simulink model "TRIAD"  (R2017a)
settings: Solver=ode4  StartTime=0.0  StopTime=20000  FixedStep=0.1  RelTol=1e-3  EnableMultiTasking=on
undefined symbols (not defined in the file): mbaseserialmask, RxBuffer
libraries: xpcseriallib x17, vrlib x7, slrtlib x4, sharedtransform x3, sharedutil x2, dspinverses x2, dspmathops x2, simulink x1, dspsigops x1
(part 2 of 3)

== system TRIAD/Subsystem/Comm and data set/Packet ZOH ==
  note: Packet Size = 22
      | =============
      | Header: 2Byte
      | Length: 1Byte
      | Time: 4 Bytes (Float32)
      | torqueX: 2Byte
      | torqueY: 2Byte
      | torqueZ: 2Byte
      | Roll      : 2Byte
      | Pitch    : 2Byte
      | Yaw     : 2Byte
      | dummy: 1byte
      | CRC: 2Byte
      | =============
  packet _count : Inport
  Data Store Write1 : DataStoreWrite  DataStoreName=RxBuffer  DataStoreElements=RxBuffer(:)
  If1 : If
  Merge1 : Merge
  No packet received Use buffer value : Subsystem  TreatAsAtomicUnit=on
  Select Main Packet : Selector  InputPortWidth=23  IndexOptions=Index vector (dialog)  Indices=[2:23]  OutputSizes=1
  Select Packet Size : Selector  InputPortWidth=23  IndexOptions=Index vector (dialog)  Indices=[1]  OutputSizes=1
  UDP Memory1 : DataStoreMemory  DataStoreName=RxBuffer  ReadBeforeWriteMsg=warning  WriteAfterWriteMsg=warning  WriteAfterReadMsg=warning  VectorParams1D=off  ShowAdditionalParam=off  Dimensions=22
  Valid Packet (Bypass) : Subsystem  TreatAsAtomicUnit=on
  packet : Outport
  wires:
  Select Main Packet/1 -> Valid Packet (Bypass)/1(In1)
  Select Packet Size/1 -> If1/1
  packet _count/1 -> Select Packet Size/1, Select Main Packet/1
  Valid Packet (Bypass)/1(Out1) -> Merge1/1
  Merge1/1 -> Data Store Write1/1, packet/1
  If1/2 -> No packet received Use buffer value/Action
  No packet received Use buffer value/1(Out1) -> Merge1/2
  If1/1 -> Valid Packet (Bypass)/Action

== system TRIAD/Subsystem10/Subsystem7/eular rotational equation2 ==
  Torque : Inport
  Inertial : Inport  Port=2
  omega_0 : Inport  Port=3
  " LU Inverse" : dspinverses/ LU Inverse
      settings: SourceProductName=DSP System Toolbox
  Cross Product : vrlib/Utilities/Cross Product
      settings: SourceProductBaseCode=VR
  Integrator1 : Integrator  InitialConditionSource=external
  Matrix Multiply : Product  Multiplication=Matrix(*)
  Matrix Multiply1 : Product  Multiplication=Matrix(*)
  Sum : Sum  Inputs=|-+
  omega : Outport
  omega_dot : Outport  Port=2
  wires:
  omega_0/1 -> Integrator1/2
  Matrix Multiply1/1 -> Integrator1/1, omega_dot/1
  Matrix Multiply/1 -> Cross Product/2
  Cross Product/1 -> Sum/1
  Torque/1 -> Sum/2
  Inertial/1 -> Matrix Multiply/1, " LU Inverse"/1
  Integrator1/1 -> Cross Product/1, Matrix Multiply/2, omega/1
  " LU Inverse"/1 -> Matrix Multiply1/1
  Sum/1 -> Matrix Multiply1/2

== system TRIAD/Subsystem10/Subsystem8/Kinematics (quaternion2)1 ==
  quat : Inport
  omega : Inport  Port=2
  Gain : Gain  Gain=0.5  SaturateOnIntegerOverflow=on  OutDataTypeStr=Inherit: Same as input  ParamDataTypeStr=Inherit: Same as input
  Mux1 : Mux  Inputs=2
  Mux2 : Mux
  q1dot : Fcn  Expr=-u(2)*u(5) - u(3)*u(6) - u(4)*u(7)
  q2dot : Fcn  Expr=u(1)*u(5) + u(3)*u(7) - u(4)*u(6)
  q3dot : Fcn  Expr=u(1)*u(6) - u(2)*u(7) + u(4)*u(5)
  q4dot : Fcn  Expr=u(1)*u(7) + u(2)*u(6) - u(3)*u(5)
  quat2dot : Outport
  wires:
  Mux2/1 -> Gain/1
  Mux1/1 -> q1dot/1, q2dot/1, q4dot/1, q3dot/1
  q1dot/1 -> Mux2/1
  q2dot/1 -> Mux2/2
  q3dot/1 -> Mux2/3
  q4dot/1 -> Mux2/4
  Gain/1 -> quat2dot/1
  quat/1 -> Mux1/1
  omega/1 -> Mux1/2

== system TRIAD/Subsystem10/Subsystem8/quat to Euler1 ==
  quat : Inport
  Mux : Mux  Inputs=3
  phi : Fcn  Expr=atan2( 2*(u(3)*u(4) + u(1)*u(2)) , u(1)^2 - u(2)^2 - u(3)^2 + u(4)^2 )
  psi : Fcn  Expr=atan2( 2*(u(2)*u(3) + u(1)*u(4)) , u(1)^2 + u(2)^2 - u(3)^2 - u(4)^2 )
  theta : Fcn  Expr=asin(2*(u(1)*u(3) - u(2)*u(4)))
  euler : Outport
  wires:
  Mux/1 -> euler/1
  phi/1 -> Mux/1
  theta/1 -> Mux/2
  psi/1 -> Mux/3
  quat/1 -> psi/1, phi/1, theta/1

== system TRIAD/Subsystem9/Subsystem7/eular rotational equation2 ==
  Torque : Inport
  Inertial : Inport  Port=2
  omega_0 : Inport  Port=3
  " LU Inverse" : dspinverses/ LU Inverse
      settings: SourceProductName=DSP System Toolbox
  Cross Product : vrlib/Utilities/Cross Product
      settings: SourceProductBaseCode=VR
  Integrator1 : Integrator  InitialConditionSource=external
  Matrix Multiply : Product  Multiplication=Matrix(*)
  Matrix Multiply1 : Product  Multiplication=Matrix(*)
  Sum : Sum  Inputs=|-+
  omega : Outport
  omega_dot : Outport  Port=2
  wires:
  omega_0/1 -> Integrator1/2
  Matrix Multiply1/1 -> Integrator1/1, omega_dot/1
  Matrix Multiply/1 -> Cross Product/2
  Cross Product/1 -> Sum/1
  Torque/1 -> Sum/2
  Inertial/1 -> Matrix Multiply/1, " LU Inverse"/1
  Integrator1/1 -> Cross Product/1, Matrix Multiply/2, omega/1
  " LU Inverse"/1 -> Matrix Multiply1/1
  Sum/1 -> Matrix Multiply1/2

== system TRIAD/Subsystem9/Subsystem8/Kinematics (quaternion2)1 ==
  quat : Inport
  omega : Inport  Port=2
  Gain : Gain  Gain=0.5  SaturateOnIntegerOverflow=on  OutDataTypeStr=Inherit: Same as input  ParamDataTypeStr=Inherit: Same as input
  Mux1 : Mux  Inputs=2
  Mux2 : Mux
  q1dot : Fcn  Expr=-u(2)*u(5) - u(3)*u(6) - u(4)*u(7)
  q2dot : Fcn  Expr=u(1)*u(5) + u(3)*u(7) - u(4)*u(6)
  q3dot : Fcn  Expr=u(1)*u(6) - u(2)*u(7) + u(4)*u(5)
  q4dot : Fcn  Expr=u(1)*u(7) + u(2)*u(6) - u(3)*u(5)
  quat2dot : Outport
  wires:
  Mux2/1 -> Gain/1
  Mux1/1 -> q1dot/1, q2dot/1, q4dot/1, q3dot/1
  q1dot/1 -> Mux2/1
  q2dot/1 -> Mux2/2
  q3dot/1 -> Mux2/3
  q4dot/1 -> Mux2/4
  Gain/1 -> quat2dot/1
  quat/1 -> Mux1/1
  omega/1 -> Mux1/2

== system TRIAD/Subsystem9/Subsystem8/quat to Euler1 ==
  quat : Inport
  Mux : Mux  Inputs=3
  phi : Fcn  Expr=atan2( 2*(u(3)*u(4) + u(1)*u(2)) , u(1)^2 - u(2)^2 - u(3)^2 + u(4)^2 )
  psi : Fcn  Expr=atan2( 2*(u(2)*u(3) + u(1)*u(4)) , u(1)^2 + u(2)^2 - u(3)^2 - u(4)^2 )
  theta : Fcn  Expr=asin(2*(u(1)*u(3) - u(2)*u(4)))
  euler : Outport
  wires:
  Mux/1 -> euler/1
  phi/1 -> Mux/1
  theta/1 -> Mux/2
  psi/1 -> Mux/3
  quat/1 -> psi/1, phi/1, theta/1

== system TRIAD/Subsystem/Comm and data set/Baseboard Serial/RS232 ISR ==
  Xmt 1 : Inport
  Xmt 2 : Inport  Port=2
  function : TriggerPort  TriggerType=function-call  VariantControl=Variant
  Demux : Demux
  Read Int Status FC1 : xpcseriallib/Mainboard/Baseboard Serial Internal  blocks/Read Int Status FC  addr1=baddr1  addr2=baddr2
      settings: SourceProductName=Simulink Real-Time  SourceProductBaseCode=XP
  Receive 1 : Subsystem  TreatAsAtomicUnit=on
  Receive 2 : Subsystem  TreatAsAtomicUnit=on
  Transmit 1 : Subsystem  TreatAsAtomicUnit=on
  Transmit 2 : Subsystem  TreatAsAtomicUnit=on
  Recv 1 : Outport
  Recv 2 : Outport  Port=2
  wires:
  Receive 1/1(Recv 1) -> Recv 1/1
  Xmt 1/1 -> Transmit 1/1(Xmt 1)
  Receive 2/1(Recv 2) -> Recv 2/1
  Xmt 2/1 -> Transmit 2/1(Xmt 2)
  Read Int Status FC1/1 -> Demux/1
  Demux/1 -> Receive 1/Trigger
  Demux/4 -> Transmit 2/Trigger
  Demux/3 -> Receive 2/Trigger
  Demux/2 -> Transmit 1/Trigger
  Read Int Status FC1/2 -> Transmit 1/2(Enable), Transmit 2/2(Enable)

== system TRIAD/Subsystem/Comm and data set/Packet ZOH/No packet received Use buffer value ==
  Action Port : ActionPort  ActionType=else
  Data Store Read : DataStoreRead  DataStoreName=RxBuffer  DataStoreElements=RxBuffer(:)
  Out1 : Outport
  wires:
  Data Store Read/1 -> Out1/1

== system TRIAD/Subsystem/Comm and data set/Packet ZOH/Valid Packet (Bypass) ==
  In1 : Inport
  Action Port : ActionPort  ActionType=then
  Out1 : Outport
  wires:
  In1/1 -> Out1/1

== system TRIAD/Subsystem/Comm and data set/Baseboard Serial/RS232 ISR/Receive 1 ==
  function : TriggerPort  TriggerType=function-call  VariantControl=Variant
  Constant : Constant  OutDataTypeStr=uint32
  FIFO write 1 : xpcseriallib/FIFO write   size=1024  inputtype=count+32 bit uint  present=off  sampletime=-1  id=RCV channel 1, IRQ 4
      settings: SourceProductName=Simulink Real-Time  SourceProductBaseCode=XP
  Read HW FIFO1 : xpcseriallib/Mainboard/Baseboard Serial Internal  blocks/Read HW FIFO  flush=on  addr=baddr1
      settings: SourceProductName=Simulink Real-Time  SourceProductBaseCode=XP
  Recv 1 : Outport
  wires:
  Read HW FIFO1/1 -> FIFO write 1/1
  FIFO write 1/1 -> Recv 1/1
  Constant/1 -> Read HW FIFO1/1

== system TRIAD/Subsystem/Comm and data set/Baseboard Serial/RS232 ISR/Receive 2 ==
  function : TriggerPort  TriggerType=function-call  VariantControl=Variant
  Constant : Constant  OutDataTypeStr=uint32
  FIFO write 2 : xpcseriallib/FIFO write   size=1024  inputtype=count+32 bit uint  present=off  sampletime=-1  id=RCV channel 2, IRQ 4
      settings: SourceProductName=Simulink Real-Time  SourceProductBaseCode=XP
  Read HW FIFO2 : xpcseriallib/Mainboard/Baseboard Serial Internal  blocks/Read HW FIFO  flush=on  addr=baddr2
      settings: SourceProductName=Simulink Real-Time  SourceProductBaseCode=XP
  Recv 2 : Outport
  wires:
  Read HW FIFO2/1 -> FIFO write 2/1
  FIFO write 2/1 -> Recv 2/1
  Constant/1 -> Read HW FIFO2/1

== system TRIAD/Subsystem/Comm and data set/Baseboard Serial/RS232 ISR/Transmit 1 ==
  Xmt 1 : Inport
  Enable : Inport  Port=2
  function : TriggerPort  TriggerType=function-call  VariantControl=Variant
  Constant1 : Constant  OutDataTypeStr=uint32
  FIFO read 1 : xpcseriallib/FIFO read   maxsize=60  minsize=1  usedelimiter=off  delimiter=13  outputtype=count+32 bit uint  enable=on  enableout=on  sampletime=-1
      settings: SourceProductName=Simulink Real-Time  SourceProductBaseCode=XP
  Write HW FIFO1 : xpcseriallib/Mainboard/Baseboard Serial Internal  blocks/Write HW FIFO  addr=baddr1
      settings: SourceProductName=Simulink Real-Time  SourceProductBaseCode=XP
  wires:
  Constant1/1 -> FIFO read 1/3
  FIFO read 1/2 -> Write HW FIFO1/2
  FIFO read 1/1 -> Write HW FIFO1/1
  Xmt 1/1 -> FIFO read 1/1
  Enable/1 -> FIFO read 1/2

== system TRIAD/Subsystem/Comm and data set/Baseboard Serial/RS232 ISR/Transmit 2 ==
  Xmt 2 : Inport
  Enable : Inport  Port=2
  function : TriggerPort  TriggerType=function-call  VariantControl=Variant
  Constant2 : Constant  OutDataTypeStr=uint32
  FIFO read 2 : xpcseriallib/FIFO read   maxsize=60  minsize=1  usedelimiter=off  delimiter=13  outputtype=count+32 bit uint  enable=on  enableout=on  sampletime=-1
      settings: SourceProductName=Simulink Real-Time  SourceProductBaseCode=XP
  Write HW FIFO2 : xpcseriallib/Mainboard/Baseboard Serial Internal  blocks/Write HW FIFO  addr=baddr2
      settings: SourceProductName=Simulink Real-Time  SourceProductBaseCode=XP
  wires:
  Constant2/1 -> FIFO read 2/3
  FIFO read 2/2 -> Write HW FIFO2/2
  FIFO read 2/1 -> Write HW FIFO2/1
  Enable/1 -> FIFO read 2/2
  Xmt 2/1 -> FIFO read 2/1

== matlab function TRIAD/Subsystem5/Keplerian Differential Equation ==
  data: kepel input; deltakep output
function deltakep  = delkep(kepel)
% [deltakep] = delkep (kep_el)
%	Function delkep calculates the rate of
%	variation of keplerian elements, considering only
%	J2 and J4.
%
% Input:
%	kep_el
% 		vector with the keplerian elements:
%		(1) - semimajor axis of the orbit in meters.
%		(2) - eccentricity.
%		(3) - inclination in radians.
%		(4) - right ascension of ascending node in radians.
%		(5) - argument of perigee in radians.
%		(6) - mean anomaly in radians.
%       Obs: 4,5 and 6 are not used
%
% Output:
%	deltakep
%		(1) = 0
%		(2) = 0
%		(3) = 0
%		(4) - variation rate of the right ascension of
%		      ascending node, in radians/second.
%		(5) - variation rate of the argument of perigee,
%			  in radians/second.
%		(6) - variation rate of the mean anomaly, in
%			  radians/second.
%
% Authors:
%	Valder M. de Medeiros  	september/81 	version 1.0
%	Valdemir Carrara 		july 2005		(C Version)
%   Valdemir Carrara            March/09        Matlab

EARTH_RADIUS	= 6378139.;				% Earth's radius in meters
EARTH_GRAVITY	= 3.9860064e+14;		% Earth's gravitational constant (m**3/s**2)
J_2 			=  1.0826268362e-3;		% = 484.16544e-6 * SQRT(5.e0)
J_4 			= -1.62336e-6;			% = -0.54112e-6 * 3e0

seix = kepel(1);
exce = kepel(2);
exc2 = exce*exce;
eta2 = 1. - exc2;
eta1 = sqrt(eta2);
teta = cos(kepel(3));
tet2 = teta*teta;
tet4 = tet2*tet2;
aux0 = sqrt(EARTH_GRAVITY/(seix*seix*seix));
plar = EARTH_RADIUS/(seix*eta2);
pla2 = plar*plar;
gam2 = 0.5*J_2*pla2;
gam4 = -0.375*J_4*pla2*pla2;

deltakep = [0, 0, 0, 0, 0, 0];

deltakep(4) = aux0*teta*(3.*gam2*(-1. + 0.125*gam2*(9.*eta2 + 12.*eta1 - ...
	   5. - (5.*eta2 + 36.*eta1 + 35.)*tet2)) + ...
	   1.25*gam4*(5. - 3.*eta2)*(3. - 7.*tet2));
deltakep(5) = aux0*(1.5*gam2*((5.*tet2 - 1.) + ...
	   0.0625*gam2*(25.*eta2 + 24.*eta1 - ...
	   35. + (90. - 192.*eta1 - 126.*eta2)*tet2 + ...
	   (385. + 360.*eta1 + 45.*eta2)*tet4)) + ...
	   0.3125*gam4*(21. - 9.*eta2 + (-270. + 126.*eta2)*tet2 + ...
	   (385. - 189.*eta2)*tet4));
deltakep(6) = aux0*(1. + eta1*(1.5*gam2*((3.*tet2 - 1.) + ...
	   0.0625*gam2*(16.*eta1 + 25.*eta2 - 15. + ...
	   (30. - 96.*eta1 - 90.*eta2)*tet2 + ...
	   (105. + 144.*eta1 + 25.*eta2)*tet4)) + ...
	   0.9375*gam4*exc2*(3. - 30.*tet2 + 35.*tet4)));

== matlab function TRIAD/Subsystem2/Convert Keplerian parameters to states ==
  data: kepel input; statvec output
function statvec = kepel_statvec(kepel)
%  [statvec] = kepel_statvec (kepel)
%	The function kepel_statvec transforms the keplerian
%	elements kepel into the corresponding state vector in
%	the same reference system.
%
% Input:
%	kepel
% 		vector containing the keplerian elements:
%		(1) - semimajor axis of the orbit in meters.
%		(2) - eccentricity.
%		(3) - inclination in radians.
%		(4) - right ascension of ascending node in radians.
%		(5) - argument of perigee in radians.
%		(6) - mean anomaly in radians.
%
% Output:
%	statvec
%  		state vector in meters and meters/second.
%
% Authors:
%	Helio K. Kuga;
%	Valder M. Medeiros;
%	Valdemir Carrara		february/80		version 1.0
%	Valdemir Carrara		july 2005		(C version)
%   Valdemir Carrara            March/09        Matlab

EARTH_GRAVITY	= 3.9860064e+14;		% Earth's gravitational constant (m**3/s**2)

a    = kepel(1);	% semi-major axis
exc  = kepel(2);	% eccentricity

c1   = sqrt(1. - exc*exc);

% Rotational matrix
rot_maz1 =  [cos(-kepel(4)), sin(-kepel(4)), 0;
             -sin(-kepel(4)), cos(-kepel(4)), 0; 
             0, 0, 1];
         
rot_max =  [1, 0, 0; 
           0, cos(-kepel(3)), sin(-kepel(3));
           0, -sin(-kepel(3)), cos(-kepel(3))];
       
rot_maz2 =  [cos(-kepel(5)), sin(-kepel(5)), 0;
             -sin(-kepel(5)), cos(-kepel(5)), 0; 
             0, 0, 1];
         
orb2iner = rot_maz1*rot_max*rot_maz2;

%%%%%%%%%%%%%%%%%%%%%%%%%%%%%%%%%%%%%%%%%%%%
%     Kepler's equation
%E    = kepler(kepel(6), exc);
mean_anomaly = kepel(6);
eccentricity = exc;
%function [eccentric] = kepler (mean_anomaly, eccentricity)
% [eccentric] = kepler (mean_anomaly, eccentricity)
%	The subroutine kepler finds a solution to the
%	kepler's equation.
%
% Input:
%	mean_anomaly
%		mean anomaly in radians.
%	eccentricity
%		eccentricity.
%
% Output:
%	eccentric
%		eccentric anomaly in radians.
%
% Authors:
%	Valder M. de Medeiros		june/81		version 2.0
%	Valdemir Carrara			july 2005	(C version)
%   Valdemir Carrara            March/09        Matlab

exc2    = eccentricity*eccentricity;
am1     = mod (mean_anomaly, 2*pi);
am2     = am1 + am1;
am3     = am1 + am2;
shoot   = am1 + eccentricity*(1. - 0.125*exc2)*sin(am1) + ...
		0.5*exc2*(sin(am2) + 0.75*eccentricity*sin(am3));
shoot   = mod (shoot, 2*pi);

e1      = 1.0;
ic      = 0;

while ((abs(e1) > 1.e-12) && (ic <= 10)) 
	e1    = (shoot - am1 - eccentricity*sin(shoot)) / ...
			(1.0 - eccentricity*cos(shoot));
    shoot = shoot - e1;
    ic    = ic + 1;
end

if (ic >= 10)
    disp ('warning ** subroutine kepler did not converge in 10 iterations');
end

%eccentric = shoot;
E = shoot;
%%%%%%%%%%%%%%%%%%%%%%%%%%%%%%%%%%%%%%%%%%%%%%
sE   = sin(E);
cE   = cos(E);
c3   = sqrt(EARTH_GRAVITY/a)/(1. - exc*cE);

%     state vector

statvec = [[a*(cE - exc), a*c1*sE, 0]*orb2iner', [-c3*sE, c1*c3*cE, 0]*orb2iner'];

== matlab function TRIAD/Ephemerides Date/Modified Julian Date (mjd) ==
  data: dmy input; diju output
function diju  =  djm (dmy)
% [diju] = djm (day, month, year)
%    The function djm furnishes the Modified Julian
%    Date with reference to the day, month and year,
%    at zero hours of the day.
% inputs:
%   dmy(1): day, day of the month
%   dmy(2): month, month of the year
%   dmy(3): year

% outputs:
%   diju
%       Modified Julian Date in days, referred to 1950.0. 
%
% Valdemir Carrara, Apr, 2003
%

diju = 367*dmy(3) + dmy(1) - 712269 + fix(275*dmy(2)/9)- fix(7*(dmy(3)+fix((dmy(2)+9)/12))/4);

== matlab function TRIAD/Ephemerides Date/Modified Julian Date (mjd0) ==
  data: dmy input; diju output
function diju  =  djm (dmy)
% [diju] = djm (day, month, year)
%    The function djm furnishes the Modified Julian
%    Date with reference to the day, month and year,
%    at zero hours of the day.
% inputs:
%   dmy(1): day, day of the month
%   dmy(2): month, month of the year
%   dmy(3): year

% outputs:
%   diju
%       Modified Julian Date in days, referred to 1950.0. 
%
% Valdemir Carrara, Apr, 2003
%

diju = 367*dmy(3) + dmy(1) - 712269 + fix(275*dmy(2)/9)- fix(7*(dmy(3)+fix((dmy(2)+9)/12))/4);

== matlab function TRIAD/Ephemerides Date/Modified Julian Date (mjd1) ==
  data: dmy input; diju output
function diju  =  djm (dmy)
% [diju] = djm (day, month, year)
%    The function djm furnishes the Modified Julian
%    Date with reference to the day, month and year,
%    at zero hours of the day.
% inputs:
%   dmy(1): day, day of the month
%   dmy(2): month, month of the year
%   dmy(3): year

% outputs:
%   diju
%       Modified Julian Date in days, referred to 1950.0. 
%
% Valdemir Carrara, Apr, 2003
%

diju = 367*dmy(3) + dmy(1) - 712269 + fix(275*dmy(2)/9)- fix(7*(dmy(3)+fix((dmy(2)+9)/12))/4);

== matlab function TRIAD/Ephemerides Time ==
  data: hours input; dayf output; minutes input; seconds input
function dayf  = time_to_dayf(hours, minutes, seconds)
% [dayf] = time_to_dayf (hours, minutes, seconds)
%    The function time_to_dayf returns with the day elapesed
%    time in seconds
% inputs:
%   hours     
%       day hour (integer).
%   minutes
%       minutes (integer).
%   seconds
%       seconds and fraction of second
% outputs:
%   dayf
%       Day elapsed time in seconds. 
%
% Valdemir Carrara, Feb, 2009
%

dayf = seconds + 60*(minutes + 60*hours);

== matlab function TRIAD/Subsystem9/MATLAB Function ==
  data: Magnetic_torque output; gyro input; Magnetic_torque input; flg output
function [Magnetic_torque, flg] = fcn(gyro, Magnetic_torque)

persistent stack_magx
persistent stack_magy
persistent stack_magz
persistent cnt_

if isempty(stack_magx)
    stack_magx = 0;
    stack_magy = 0;
    stack_magz = 0;
    cnt_ = 0;
else
    cnt_ = cnt_ + 1;
end

flg = 0;

if cnt_ >= 100
    if (abs(stack_magx)<0.1) && (abs(stack_magy)<0.1) && (abs(stack_magz)<0.1)
        flg = 1;
        Magnetic_torque = [0 0 0]';
    else
        flg = 0;
    end
    stack_magx = 0;
    stack_magy = 0;
    stack_magz = 0;
    cnt_ = 0;
else
    stack_magx = stack_magx + gyro(1);
    stack_magy = stack_magy + gyro(2);
    stack_magz = stack_magz + gyro(3);
end



end

== matlab function TRIAD/Subsystem2/ECI to ECEF  ==
  data: tesig input; xterrestrial output; xi input
function xterrestrial  = inertial_to_terrestrial (tesig, xi)
% [xterrestrial] = inertial_to_terrestrial (tesig, xi)
%	The function inertial_to_terrestrial transforms geocentric
%	inertial state vector into geocentric
%	terrestrial coordinates (referred to
%	Greenwich).
%
% Input:
%	tesig
%		Greenwich sidereal time in radians.
%	xi
%		geocentric inertial position vector.
%       (1) inertial geocentric position x (m)
%       (2) inertial geocentric position y (m)
%       (3) inertial geocentric position z (m)
%       (4) inertial geocentric velocity x (m/s)
%       (5) inertial geocentric velocity y (m/s)
%       (6) inertial geocentric velocity z (m/s)
%
% Output:
%	xterrestrial
%		corresponding geocentric terrestrial vector.
%
% Authors:
%	Helio/Valder/Valdemir-aug. 1981 - version 1.0
%	Helio		-july 1989 - version 1.1
%	Valdemir Carrara		july 2005		(C version)
%   Valdemir Carrara            March/09        Matlab
coan    =  cos(tesig);
sian    =  sin(tesig);
rot_mat =  [ coan, sian, 0 ;
            -sian, coan, 0 ; 
                0,    0, 1];

xterrestrial_ = [xi(1:3); xi(4:6)]*rot_mat';
xterrestrial  = [xterrestrial_(1,:) xterrestrial_(2,:)];

== matlab function TRIAD/Subsystem2/Convert Terrestrial Geocentric to Speherical coordinates ECEF2LLA ==
  data: geoc input; spherical output
function spherical  = rectangular_to_spherical (geoc)
% [spherical] = rectangular_to_spherical (geoc)
%	Function to transform rectangular terrestrial
%	geocentric coordinates in spherical coordinates
%	(longitude, geocentric latitude and distance).
%
% Inputs:
%   geoc
%   		geocentric rectangular coordinates vector in meters
%           (1) geocentric position x (m)
%           (2) geocentric position y (m)
%           (3) geocentric position z (m)
%
% Outputs:
%	spherical
%		Geocentric coordinates vector:
%			1 = east longitude (rad)
%			2 = geocentric latitude (rad)
%			3 = geocentric distance (meters)
%
% Authors:
%   Valdemir Carrara            May/09        Matlab

px = geoc(1);
py = geoc(2);
pz = geoc(3);
ws = px*px + py*py;
rw = sqrt(ws + pz *pz);
lg = atan2(py, px);
lt = atan2(pz, sqrt(ws));
spherical = [lg, lt, rw];

== matlab function TRIAD/Greenwich Aparent Mean Sideral Time ==
  data: diju input; gwst output; time input
function gwst  = gst (diju, time)
% [gwst] = gst (diju, time)
%   The function gst furnishes the greenwich aparent mean 
%   sidereal time referred to the J2000.0 equator and equinox.
% inputs:
%   diju
%       Modified Julian Date in days, referred to 1950.0.
%   time
%       UT1 time complement in seconds.
% outputs:
%   gwst
%       Greenwich aparent sidereal time in radians
%
% Valdemir Carrara, Apr, 2003
%

tsj = (diju-18262.5)/36525;
tsgo = (24110.54841 + (8640184.812866 + 9.3104e-2*tsj - 6.2e-6*tsj*tsj)*tsj)*pi/43200;
tetp = 7.292116e-5;		% velocidade angular da Terra (rd/s) mean angular velocity of the Earth
gwst = mod(tsgo + time*tetp, 2*pi);
% reference site
% https://www2.mps.mpg.de/homes/fraenz/systems/systems2art/node10.html
%      if (gwst<0) gwst = gwst + 2*pi

== matlab function TRIAD/Subsystem4/Compute IGRF Field ==
  data: time input; B output; latitude input; longitude input; altitude input
function B    = igrf12(time, latitude, longitude, altitude)
% IGRF 12 Calculation
% For Geocentric spherical coordinates
% Written by Thomas Jung
% Date: 2017. 7. 9
% Extracted code from Matlab igrf.m

% For index 24 (2015)
lastgh = [-29442.0,  -1501.0,    4797.1, -2445.1,    3012.9, -2845.6,    1676.7, -641.9, ...
        1350.7,     -2352.3,    -115.3, 1225.6,     244.9,  582.0,      -538.4, 907.6,  ...
        813.7,      283.3,      120.4,  -188.7,     -334.9, 180.9,      70.4,   -329.5, ...
       -232.6,      360.1,      47.3,   192.4,      197.0,  -140.9,     -119.3, -157.5, ...
         16.0,      4.1,        100.2,  70.0,       67.7,   -20.8,      72.7,   33.2, ...
       -129.9,      58.9,       -28.9,  -66.7,      13.2,   7.3,        -70.9,  62.6, ...
         81.6,      -76.1,      -54.1,  -6.8,       -19.5,  51.8,       5.7,    15.0, ...
         24.4,      9.4,        3.4,    -2.8,       -27.4,  6.8,        -2.2,   24.2, ...
          8.8,      10.1,       -16.9,  -18.3,      -3.2,   13.3,       -20.6,  -14.6, ...
         13.4,      16.2,       11.7,   5.7,        -15.9,  -9.1,       -2.0,   2.1, ...
          5.4,      8.8,        -21.6,  3.1,        10.8,   -3.3,       11.8,   0.7, ...
         -6.8,      -13.3,      -6.9,   -0.1,       7.8,    8.7,        1.0,    -9.1, ...
         -4.0,      -10.5,      8.4,    -1.9,       -6.3,   3.2,        0.1,    -0.4, ...
           0.5,     4.6,        -0.5,   4.4,        1.8,    -7.9,       -0.7,   -0.6, ...
          2.1,      -4.2,       2.4,    -2.8,       -1.8,   -1.2,       -3.6,   -8.7, ...
          3.1,      -1.5,       -0.1,   -2.3,       2.0,    2.0,        -0.7,   -0.8, ...
         -1.1,      0.6,        0.8,    -0.7,       -0.2,   0.2,        -2.2,   1.7, ...
         -1.4,      -0.2,       -2.5,   0.4,        -2.0,   3.5,        -2.4,   -1.9, ...
          -0.2,     -1.1,       0.4,    0.4,        1.2,    1.9,        -0.8,   -2.2, ...
           0.9,     0.3,        0.1,    0.7,        0.5,    -0.1,       -0.3,   0.3, ...
          -0.4,     0.2,        0.2,    -0.9,       -0.9,   -0.1,       0,      0.7, ...
           0,       -0.9,       -0.9,   0.4,        0.4,    0.5,        1.6,    -0.5, ...
          -0.5,     1.0,        -1.2,   -0.2,       -0.1,   0.8,        0.4,    -0.1, ...
          -0.1,     0.3,        0.4,    0.1,        0.5,    0.5,        -0.3,   -0.4, ...
          -0.4,     -0.3,       -0.8];
% For index 25 (2020)      
nextgh = [10.3,      18.1,       -26.6,  -8.7,       -3.3,   -27.4,      2.1,    -14.1, ...
        3.4,        -5.5,       8.2,    -0.7,       -0.4,   -10.1,      1.8,    -0.7, ...
        0.2,        -1.3,       -9.1,   5.3,        4.1,    2.9,        -4.3,   -5.2, ...
        -0.2,       0.5,        0.6,    -1.3,       1.7,    -0.1,       -1.2,   1.4, ...
        3.4,        3.9,        0,      -0.3        -0.1,    0,         -0.7,   -2.1, ...
        2.1,        -0.7,       -1.2,   0.2,        0.3,    0.9,        1.6,    1.0, ...
        0.3,        -0.2,       0.8,    -0.5,       0.4,    1.3,        -0.2,   0.1, ...
        -0.3,       -0.6,       -0.6,   -0.8,       0.1,    0.2,        -0.2,   0.2, ...
        0,          -0.3,       -0.6,   0.3,        0.5,    0.1,        -0.2,   0.5, ...
        0.4,        -0.2,       0.1,    -0.3,       -0.4,   0.3,        0.3,    0, ...
        0,          0,          0,      0,          0,      0,          0,      0, ...
        0,          0,          0,      0,          0,      0,          0,      0, ...
        0,          0,          0,      0,          0,      0,          0,      0, ...
        0,          0,          0,      0,          0,      0,          0,      0, ...
        0,          0,          0,      0,          0,      0,          0,      0, ...
        0,          0,          0,      0,          0,      0,          0,      0, ...
        0,          0,          0,      0,          0,      0,          0,      0, ...
        0,          0,          0,      0,          0,      0,          0,      0, ...
        0,          0,          0,      0,          0,      0,          0,      0, ...
        0,          0,          0,      0,          0,      0,          0,      0, ...
        0,          0,          0,      0,          0,      0,          0,      0, ...
        0,          0,          0,      0,          0,      0,          0,      0, ...
        0,          0,          0,      0,          0,      0,          0,      0, ...
        0,          0,          0,      0,          0,      0,          0,      0, ...
        0,          0,          0];

ghslope = nextgh;
% years(lastepoch) = 2015
%gh = lastgh + ghslope*(time - years(lastepoch));
gh = lastgh + ghslope*(time - 2015);

% Fundamental constant.
Rearth_km = 6371.2;

%%% SPHERICAL COORDINATE CONVERSION %%%
% Convert the latitude, longitude, and altitude coordinates input into
% spherical coordinates r (radius), theta (inclination angle from +z axis),
% and phi (azimuth angle from +x axis).
% We want cos(theta) and sin(theta) rather than theta itself.
costheta = cos(pi/2 - latitude);
sintheta = sin(pi/2 - latitude);

% geocentric coordinates (chosen).
r = altitude;
cd = 1;
sd = 0;

% Convert longitude to radians.
phi = longitude;

%%% GET PROPER IGRF COEFFICIENTS %%%
ghslope = nextgh;
% years(lastepoch) = 2015
%gh = lastgh + ghslope*(time - years(lastepoch));
gh = lastgh + ghslope*(time - 2015);

nmax = sqrt(numel(gh) + 1) - 1;
% nmax should be an integer.
if nmax - round(nmax) ~= 0
    error('igrf:timeInputInvalid', ['TIME input should either be ' ...
            'a single date or a valid coefficient vector.']);
end

% We need cos(m*phi) and sin(m*phi) multiple times, so precalculate into a
% vector here:
cosphi = cos((1:nmax)*phi);
sinphi = sin((1:nmax)*phi);

Pmax = (nmax+1)*(nmax+2)/2;

%%% BEGIN MAGNETIC FIELD CALCULATION %%%
% Initialize variables used in for loop below.
Br = 0; Bt = 0; Bp = 0;
 P = zeros(1, Pmax);  P(1) = 1;  P(3) = sintheta;
dP = zeros(1, Pmax); dP(1) = 0; dP(3) = costheta;

% For this initial condition, the first if will result in n = 1, m = 0.
m = 1; n = 0; coefindex = 1;

a_r = (Rearth_km/r)^2;

% Increment through all the n's and m's. gh will be a vector with g
% followed by h for incrementing through n and m except when h would be
% redundant (i.e., when m = 0).
for Pindex = 2:Pmax
    
    % Increment to the next n when m becomes larger than n.
    if n < m
        m = 0;
        n = n + 1;
        a_r = a_r*(Rearth_km/r); % We need (Rearth_km./r)^(n+2)
    end
    
    % Calculate P and dP. They are given recursively according to:
    % 
    % P(0, 0) = 1, P(1, 1) = sin(theta) <- Specified above
    % P(n, n) = sqrt(1 - 1/(2n))*sin(theta)*P(n-1, n-1)
    % P(n, m) = (2n - 1)/sqrt(n^2 - m^2)*cos(theta)*P(n-1, m) -
    %     sqrt(((n-1)^2 - m^2) / (n^2 - m^2)) * P(n-2, m)
    % 
    % dP(0, 0) = 0, dP(1, 1) = cos(theta) <- Specified above
    % dP(n, n) = sqrt(1 - 1/(2n))*(sin(theta)*dP(n-1, n-1) +
    %     cos(theta)*P(n-1, n-1))
    % dP(n, m) = (2n - 1)/sqrt(n^2 - m^2)*(cos(theta)*dP(n-1, m) -
    %     sin(theta)*P(n-1, m)) - sqrt(((n-1)^2 - m^2)/(n^2 - m^2))*
    %     dP(n-2, m)
    if m < n && Pindex ~= 3 % (Pindex=3 is n=1, m=1, initial cond. above)
        last1n = Pindex - n;
        last2n = Pindex - 2*n + 1;
        P(Pindex) = (2*n - 1)/sqrt(n^2 - m^2)*costheta*P(last1n) - ...
            sqrt(((n-1)^2 - m^2) / (n^2 - m^2)) * P(last2n);
        dP(Pindex) = (2*n - 1)/sqrt(n^2 - m^2)*(costheta*dP(last1n) - ...
            sintheta*P(last1n)) - sqrt(((n-1)^2 - m^2) / (n^2 - m^2)) * ...
            dP(last2n);
    elseif Pindex ~= 3
        lastn = Pindex - n - 1;
        P(Pindex) = sqrt(1 - 1/(2*m))*sintheta*P(lastn);
        dP(Pindex) = sqrt(1 - 1/(2*m))*(sintheta*dP(lastn) + ...
            costheta*P(lastn));
    end
    
    % Calculate the magnetic field components as a running sum. Find
    % explicit expressions for these in Global Earth Physics: a Handbook of
    % Physical Constants by Thomas J. Aherns (1995), pg. 49. Link:
    % http://books.google.com/books?id=aqjU_NHyre4C&lpg=PP1&dq=Global%20
    % earth%20physics%3A%20a%20handbook%20of%20physical%20constants&pg=PA49
    % #v=onepage&q&f=false
    % (except equation 6 is missing a required 1/sin(theta) and m; correct
    % equations on page 5 (equations 3a-3c) of:
    % http://hanspeterschaub.info/Papers/UnderGradStudents/
    % MagneticField.pdf)
    if m == 0 % Implies h = 0, so only coefficient in gh is g
        coef = a_r*gh(coefindex); %*cos(0*phi) = 1
        Br = Br + (n+1)*coef*P(Pindex);%x
        Bt = Bt - coef*dP(Pindex);%z
        % Bp is 0 for m = 0.
        coefindex = coefindex + 1; % Only need to skip over g this time.
    else
        coef = a_r*(gh(coefindex)*cosphi(m) + gh(coefindex+1)*sinphi(m));
        Br = Br + (n+1)*coef*P(Pindex);
        Bt = Bt - coef*dP(Pindex);
        if sintheta == 0 % Use different formula when dividing by 0.
            Bp = Bp - costheta*a_r*(-gh(coefindex)*sinphi(m) + ...
                gh(coefindex+1)*cosphi(m))*dP(Pindex);
        else
            Bp = Bp - 1/sintheta*a_r*m*(-gh(coefindex)*sinphi(m) + ...
                gh(coefindex+1)*cosphi(m))*P(Pindex);
        end
        coefindex = coefindex + 2; % Skip over g and h this time.
    end
    
    % Increment m.
    m = m + 1;
    
end

% Convert from spherical to (x,y,z) = (North,East,Down).
Bx = -Bt;
By = Bp;
Bz = -Br;
% Convert back to geodetic coordinates if necessary.
Bx_old = Bx;
Bx = Bx.*cd + Bz.*sd;
Bz = Bz.*cd - Bx_old.*sd;

B = [Bx; By; Bz];
end

== matlab function TRIAD/Subsystem4/Subsystem/Rotation matrix (ECEF to NED) ==
  data: mat output; lat input; lon input
function mat   = ECEF2NED(lat, lon)
% https://kr.mathworks.com/help/aeroblks/directioncosinematrixeceftoned.html
% [my_ned2ecef( n, e, d, lat, lon, alt )]
% lat, lon  : rad
    R1 = [-sin(lat), 0, cos(lat);
               0   , 1,    0    ;
          -cos(lat), 0,-sin(lat)
          ];
    R2 = [ cos(lon), sin(lon), 0;
          -sin(lon), cos(lon), 0;
               0   ,    0    , 1
         ];
    mat = R1 * R2; % This is DCM (From ECEF to NED)
    mat = mat';    % Convert to Rotation matrix
end

== matlab function TRIAD/Subsystem4/Subsystem/Rotation matrix (ECI to ECEF) ==
  data: GMST input; mat output
function mat  = eci2ecef(GMST)

GMST  = rem(GMST,2*pi);

sGMST = sin(GMST);
cGMST = cos(GMST);

ROT_Z   = [      cGMST,  -1*sGMST, 0; 
                 sGMST,    cGMST , 0; 
                   0  ,      0   , 1];
mat =  ROT_Z;
              
end

== matlab function TRIAD/Subsystem4/Subsystem/Rotation matrix (ECI to Perifocal) ==
  data: ke input; mat output
function mat = eci2perifocal( ke )
RAAN         = ke(4,1);%rem(ke(4,1),2*pi)
Arg_perigee  = ke(5,1);%rem(ke(5,1),2*pi)
inclination  = ke(3,1);%rem(ke(3,1),2*pi);

% theta1 = (RAAN + Arg_perigee);%rem((RAAN + Arg_perigee),2*pi);
R1 = [   cos(RAAN),  -sin(RAAN), 0;
            sin(RAAN),   cos(RAAN), 0;
                 0     ,          0     , 1 ];
             
R2 = [      1,          0    ,           0;
            0,     cos(inclination),    -sin(inclination);
            0,     sin(inclination),       cos(inclination)];
        
R3 = [   cos(Arg_perigee),  -sin(Arg_perigee), 0;
            sin(Arg_perigee),     cos(Arg_perigee), 0;
                 0     ,          0     , 1];
             
mat = R1 * R2 * R3;
end

== matlab function TRIAD/Subsystem4/Subsystem/Rotation matrix (Perifocal to Orbit) ==
  data: ke input; mat output
function mat = perifocal2orbit( ke )
% 		vector with the keplerian elements:
%		(1) - semimajor axis of the orbit in meters.
%		(2) - eccentricity.
%		(3) - inclination in radians.
%		(4) - right ascension of ascending node in radians.
%		(5) - argument of perigee in radians.
%		(6) - mean anomaly in radians.
mean_anomaly = ke(6,1);
%theta = rem(mean_anomaly,2*pi);

R1 = [ cos(mean_anomaly + pi/2),-sin(mean_anomaly + pi/2), 0;
       sin(mean_anomaly + pi/2), cos(mean_anomaly + pi/2), 0;
             0        ,         0        , 1    ];
R2 = [  1,     0     ,      0     ; 
        0, cos(-pi/2), -sin(-pi/2);
        0, sin(-pi/2),  cos(-pi/2)];

mat = R1 * R2;

end

== matlab function TRIAD/Subsystem9/MATLAB Function1 ==
  data: mag_delay input; B_dot output; mag input
function B_dot = fcn(mag_delay, mag)
B_dot = (mag_delay - mag)/1;
end

== matlab function TRIAD/Subsystem9/MATLAB Function5 ==
  data: torque_in input; torque_out output; logic input
function torque_out = fcn(torque_in, logic)

t_x = torque_in(1,1);
t_y = torque_in(2,1);
t_z = torque_in(3,1);

if logic == 0
    torque_out = [t_x,t_y,t_z]';
else
    torque_out = [0,0,0]';
end

end

== matlab function TRIAD/Subsystem9/MATLAB Function6 ==
  data: torque_in input; torque_out output; logic input
function torque_out = fcn(torque_in, logic)

t_x = torque_in(1,1);
t_y = torque_in(2,1);
t_z = torque_in(3,1);

if logic == 0
    torque_out = [t_x,t_y,t_z]';
else
    torque_out = [0,0,0]';
end

end

== matlab function TRIAD/Subsystem9/Smoothing ==
  data: B_dotf input; B_dotmb input; B_dotm output
function B_dotm = fcn(B_dotf,B_dotmb)
%#codegen
s=0.5;
B_dotm = (1-s)*B_dotf + s*B_dotmb;

== matlab function TRIAD/Subsystem9/MATLAB Function12 ==
  data: moment input; Trans_moment output
function Trans_moment = fcn(moment)
    
%     moment_temp_x = 0;  moment_temp_y = 0;  moment_temp_z = 0;
%     Trans_moment = zeros(3,1);
%     
%     moment_temp_x   =   moment(1,1) * 68420;
%     moment_temp_y   =   moment(2,1) * 68420;
%     moment_temp_z   =   moment(3,1) * 68420;
%     
%     if(moment_temp_x < -0.2)
%         Trans_moment(1,1) = -0.2/68420;
%     elseif(moment_temp_x > 0.2)
%         Trans_moment(1,1) = 0.2/68420;
%     end
% 
%     if(moment_temp_y < -0.2)
%         Trans_moment(2,1) = -0.2/68420;
%     elseif(moment_temp_y > 0.2)
%         Trans_moment(2,1) = 0.2/68420;
%     end
% 
%     if(moment_temp_z < -0.2)
%         Trans_moment(3,1) = -0.2/68420;
%     elseif(moment_temp_z > 0.2)
%         Trans_moment(3,1) = 0.2/68420;
%     end

    Trans_moment = zeros(3,1);
    
    moment_temp_x   =   moment(1,1);
    moment_temp_y   =   moment(2,1);
    moment_temp_z   =   moment(3,1);
    
    if(moment_temp_x < -0.1675)
        Trans_moment(1,1) = -0.1675;
    elseif(moment_temp_x > 0.1675)
        Trans_moment(1,1) = 0.1675;
    else
        Trans_moment(1,1) = moment_temp_x;
    end

    if(moment_temp_y < -0.1703 )
        Trans_moment(2,1) = -0.1703;
    elseif(moment_temp_y > 0.1703)
        Trans_moment(2,1) = 0.1703;
    else
        Trans_moment(2,1) = moment_temp_y;
    end

    if(moment_temp_z < -0.1582)
        Trans_moment(3,1) = -0.1582;
    elseif(moment_temp_z > 0.1582)
        Trans_moment(3,1) = 0.1582;
    else
        Trans_moment(3,1) = moment_temp_z;
    end

end

== matlab function TRIAD/SUN_function/Subsystem2/MATLAB Function8 ==
  data: vec input; azimuth_rad output
function azimuth_rad = fcn(vec)
x = vec(1,1);   y = vec(2,1);   z = vec(3,1);

if ( x < 0 && y == 0 && z ~= 0)
    azimuth_rad = pi;
elseif( x > 0 && y == 0 && z ~= 0)
    azimuth_rad = 0;
elseif( x == 1 && y == 0 && z == 0)
    azimuth_rad = 0;
elseif( x == 0 && y == 1 && z == 0)
    azimuth_rad = pi/2;
elseif( x == 0 && y == 0 && z == 1)
    azimuth_rad = 0;
else
    azimuth_rad = atan2(y,x);
end

end

== matlab function TRIAD/SUN_function/Subsystem2/MATLAB Function9 ==
  data: vec input; elevation output; z output
function [elevation,z] = fcn(vec)

x = vec(1,1);   y = vec(2,1);   z = vec(3,1);
temp = sqrt(x*x + y*y);

if z < 0
    elevation = -1*atan2(abs(z),temp);
elseif z >= 0
    elevation =  1*atan2(abs(z),temp);
else
    elevation = NaN;
end

end

== matlab function TRIAD/Subsystem/Comm and data set/Build binary packet ==
  data: time input; message output; muxindex input; data input
function message = build_packet_crc (time,  muxindex,  data)
% Building a packet with appended crc-ccitt16 
% Input variables
%    - time [double] : timer counter value (increment +1)
%    - muxindex [double]: Rolling data index
%    - data [double]: Actual data

% Message size
N = 44;

% Inialize the message buffer
message = uint8(zeros(N,1));

% Header : 2 bytes
message(1,:) = hex2dec('7E');
message(2,:) = hex2dec('81');

% Length : unsigned 1 bytes
message(3,:) = N;

% Time : unsigned 4 bytes
dummy = TxUint32(time);
message(4,:) = dummy(1,:);
message(5,:) = dummy(2,:);
message(6,:) = dummy(3,:);
message(7,:) = dummy(4,:);

% Longitude : signed 4 bytes
dummy = TxInt32(data(1)); %longitude_
message(8,:)  = dummy(1,:);
message(9,:)  = dummy(2,:);
message(10,:) = dummy(3,:);
message(11,:) = dummy(4,:);

% Latitude : signed 4 bytes
dummy = TxInt32(data(2));%latitude_
message(12,:) = dummy(1,:);
message(13,:) = dummy(2,:);
message(14,:) = dummy(3,:);
message(15,:) = dummy(4,:);

% Altitude : signed 4 bytes
dummy = TxInt32(data(3));%height_
message(16,:) = dummy(1,:);
message(17,:) = dummy(2,:);
message(18,:) = dummy(3,:);
message(19,:) = dummy(4,:);

% Year : signed 2 bytes
dummy = TxInt16(data(4));%year
message(20,:) = dummy(1,:);
message(21,:) = dummy(2,:);

% Month : signed 1 bytes
message(22,:) = uint8(data(5));%month

% Day : signed 1 bytes
message(23,:) = uint8(data(6));%day

% Gyrox : signed 2 bytes
dummy = TxInt16(data(7));%gyro_x
message(24,:) = dummy(1,:);
message(25,:) = dummy(2,:);

% Gyroy : signed 2 bytes
dummy = TxInt16(data(8));%gyro_y
message(26,:) = dummy(1,:);
message(27,:) = dummy(2,:);

% Gyrox : signed 2 bytes
dummy = TxInt16(data(9));%gyro_z
message(28,:) = dummy(1,:);
message(29,:) = dummy(2,:);

% Magx : signed 2 bytes
dummy = TxInt16(data(10));%mag_x
message(30,:) = dummy(1,:);
message(31,:) = dummy(2,:);

% Magy : signed 2 bytes
dummy = TxInt16(data(11));%mag_y
message(32,:) = dummy(1,:);
message(33,:) = dummy(2,:);

% Magz : signed 2 bytes
dummy = TxInt16(data(12));%mag_z
message(34,:) = dummy(1,:);
message(35,:) = dummy(2,:);

% Sunx : signed 2 bytes
dummy = TxInt16(data(13));%sun_azi
message(36,:) = dummy(1,:);
message(37,:) = dummy(2,:);

% Suny : signed 2 bytes
dummy = TxInt16(data(14));%sun_elev
message(38,:) = dummy(1,:);
message(39,:) = dummy(2,:);

% dummy = TxInt16(data(15));%sun_z
% message(40,:) = dummy(1,:);
% message(41,:) = dummy(2,:);

message(40,:) = uint8(data(15)); % hour
message(41,:) = uint8(data(16)); % minute
message(42,:) = uint8(data(17)); % sec

% Now compute the CRC-CCITT16
crc = uint16(0);

for i=3:N-2
    crc = UpdateCRC(crc, message(i,:));
end

% Finally append the crc (two bytes) at the trailer
message(43,:) = uint8(bitand(bitshift(crc, -8, 'uint16'), hex2dec('00FF')));
message(44,:) = uint8(bitand(crc, hex2dec('00FF')));
end

function Out = TxUint16(data)
Out = uint8(zeros(2,1));
Out(1,:) = bitand(bitshift(uint16(data), -8, 'uint16'), hex2dec('00FF'));
Out(2,:) = bitand(uint16(data), hex2dec('00FF'));
end

function Out = TxInt16(data)
Out = uint8(zeros(2,1));
Out(1,:) = bitand(bitshift(int16(data), -8, 'int16'), hex2dec('00FF'));
Out(2,:) = bitand(int16(data), hex2dec('00FF'));
end

function Out = TxUint32(data)
Out = uint8(zeros(4,1));
Out(1,:) = bitand(bitshift(uint32(data), -24, 'uint32'), hex2dec('000000FF'));
Out(2,:) = bitand(bitshift(uint32(data), -16, 'uint32'), hex2dec('000000FF'));
Out(3,:) = bitand(bitshift(uint32(data),  -8, 'uint32'), hex2dec('000000FF'));
Out(4,:) = bitand(uint32(data), hex2dec('000000FF'));
end

function Out = TxInt32(data)
Out = uint8(zeros(4,1));
Out(1,:) = bitand(bitshift(int32(data), -24, 'int32'), hex2dec('000000FF'));
Out(2,:) = bitand(bitshift(int32(data), -16, 'int32'), hex2dec('000000FF'));
Out(3,:) = bitand(bitshift(int32(data),  -8, 'int32'), hex2dec('000000FF'));
Out(4,:) = bitand(int32(data), hex2dec('000000FF'));
end

function crc_out = UpdateCRC(crc, bytedata)
crc_table = uint16( hex2dec( [
	'0000'; '1021'; '2042'; '3063'; '4084'; '50a5'; '60c6'; '70e7';
	'8108'; '9129'; 'a14a'; 'b16b'; 'c18c'; 'd1ad'; 'e1ce'; 'f1ef';
	'1231'; '0210'; '3273'; '2252'; '52b5'; '4294'; '72f7'; '62d6';
	'9339'; '8318'; 'b37b'; 'a35a'; 'd3bd'; 'c39c'; 'f3ff'; 'e3de';
	'2462'; '3443'; '0420'; '1401'; '64e6'; '74c7'; '44a4'; '5485';
	'a56a'; 'b54b'; '8528'; '9509'; 'e5ee'; 'f5cf'; 'c5ac'; 'd58d';
	'3653'; '2672'; '1611'; '0630'; '76d7'; '66f6'; '5695'; '46b4';
	'b75b'; 'a77a'; '9719'; '8738'; 'f7df'; 'e7fe'; 'd79d'; 'c7bc';
	'48c4'; '58e5'; '6886'; '78a7'; '0840'; '1861'; '2802'; '3823';
	'c9cc'; 'd9ed'; 'e98e'; 'f9af'; '8948'; '9969'; 'a90a'; 'b92b';
	'5af5'; '4ad4'; '7ab7'; '6a96'; '1a71'; '0a50'; '3a33'; '2a12';
	'dbfd'; 'cbdc'; 'fbbf'; 'eb9e'; '9b79'; '8b58'; 'bb3b'; 'ab1a';
	'6ca6'; '7c87'; '4ce4'; '5cc5'; '2c22'; '3c03'; '0c60'; '1c41';
	'edae'; 'fd8f'; 'cdec'; 'ddcd'; 'ad2a'; 'bd0b'; '8d68'; '9d49';
	'7e97'; '6eb6'; '5ed5'; '4ef4'; '3e13'; '2e32'; '1e51'; '0e70';
	'ff9f'; 'efbe'; 'dfdd'; 'cffc'; 'bf1b'; 'af3a'; '9f59'; '8f78';
	'9188'; '81a9'; 'b1ca'; 'a1eb'; 'd10c'; 'c12d'; 'f14e'; 'e16f';
	'1080'; '00a1'; '30c2'; '20e3'; '5004'; '4025'; '7046'; '6067';
	'83b9'; '9398'; 'a3fb'; 'b3da'; 'c33d'; 'd31c'; 'e37f'; 'f35e';
	'02b1'; '1290'; '22f3'; '32d2'; '4235'; '5214'; '6277'; '7256';
	'b5ea'; 'a5cb'; '95a8'; '8589'; 'f56e'; 'e54f'; 'd52c'; 'c50d';
	'34e2'; '24c3'; '14a0'; '0481'; '7466'; '6447'; '5424'; '4405';
	'a7db'; 'b7fa'; '8799'; '97b8'; 'e75f'; 'f77e'; 'c71d'; 'd73c';
	'26d3'; '36f2'; '0691'; '16b0'; '6657'; '7676'; '4615'; '5634';
	'd94c'; 'c96d'; 'f90e'; 'e92f'; '99c8'; '89e9'; 'b98a'; 'a9ab';
	'5844'; '4865'; '7806'; '6827'; '18c0'; '08e1'; '3882'; '28a3';
	'cb7d'; 'db5c'; 'eb3f'; 'fb1e'; '8bf9'; '9bd8'; 'abbb'; 'bb9a';
	'4a75'; '5a54'; '6a37'; '7a16'; '0af1'; '1ad0'; '2ab3'; '3a92';
	'fd2e'; 'ed0f'; 'dd6c'; 'cd4d'; 'bdaa'; 'ad8b'; '9de8'; '8dc9';
	'7c26'; '6c07'; '5c64'; '4c45'; '3ca2'; '2c83'; '1ce0'; '0cc1';
	'ef1f'; 'ff3e'; 'cf5d'; 'df7c'; 'af9b'; 'bfba'; '8fd9'; '9ff8';
	'6e17'; '7e36'; '4e55'; '5e74'; '2e93'; '3eb2'; '0ed1'; '1ef0';
]));

datain  = bitand(uint16(bytedata), hex2dec('00FF'));
crcidx  = bitxor(bitshift(crc, -8, 'uint16'), datain, 'uint16');
crcidx_temp = bitand(crcidx, hex2dec('00FF'), 'uint16');
crc_out = bitxor(bitshift(crc, 8, 'uint16'), crc_table(crcidx_temp+1), 'uint16');
end

== matlab function TRIAD/Subsystem1/MATLAB Function1 ==
  data: orbit_x input; v_orbit output; orbit_y input; orbit_z input; ecef_v input
function v_orbit  = fcn(orbit_x,orbit_y,orbit_z,ecef_v)
v_orbit = zeros(1,3);

v_orbit(1,1) = dot(ecef_v' , (orbit_x / norm(orbit_x)));
v_orbit(1,2) = dot(ecef_v' , (orbit_y / norm(orbit_y)));
v_orbit(1,3) = dot(ecef_v' , (orbit_z / norm(orbit_z)));
end

== matlab function TRIAD/Subsystem/Comm and data set/Parse binary packet (ADCS) ==
  data: packet input; data output
function data = parse_packet_crc (packet)
% Parse a packet into array with CRC Error check
% Input variables
%    - packet [uint16] : count + data
% Output variables
%    - data(1) [uint8]: Length
%    - data(2) [float32]: Time (Pixhawk time)
%    - data(3) [int16]: magnetic momentum X
%    - data(4) [int16]: magnetic momentum Y
%    - data(5) [int16]: magnetic momentum Z
%    - data(6) [int16]: TRIAD angle X
%    - data(7) [int16]: TRIAD angle Y
%    - data(8) [int16]: TRIAD angle Z
%    - data(9) [int8]: Dummy



crc_table = uint16( hex2dec( [
	'0000'; '1021'; '2042'; '3063'; '4084'; '50a5'; '60c6'; '70e7';
	'8108'; '9129'; 'a14a'; 'b16b'; 'c18c'; 'd1ad'; 'e1ce'; 'f1ef';
	'1231'; '0210'; '3273'; '2252'; '52b5'; '4294'; '72f7'; '62d6';
	'9339'; '8318'; 'b37b'; 'a35a'; 'd3bd'; 'c39c'; 'f3ff'; 'e3de';
	'2462'; '3443'; '0420'; '1401'; '64e6'; '74c7'; '44a4'; '5485';
	'a56a'; 'b54b'; '8528'; '9509'; 'e5ee'; 'f5cf'; 'c5ac'; 'd58d';
	'3653'; '2672'; '1611'; '0630'; '76d7'; '66f6'; '5695'; '46b4';
	'b75b'; 'a77a'; '9719'; '8738'; 'f7df'; 'e7fe'; 'd79d'; 'c7bc';
	'48c4'; '58e5'; '6886'; '78a7'; '0840'; '1861'; '2802'; '3823';
	'c9cc'; 'd9ed'; 'e98e'; 'f9af'; '8948'; '9969'; 'a90a'; 'b92b';
	'5af5'; '4ad4'; '7ab7'; '6a96'; '1a71'; '0a50'; '3a33'; '2a12';
	'dbfd'; 'cbdc'; 'fbbf'; 'eb9e'; '9b79'; '8b58'; 'bb3b'; 'ab1a';
	'6ca6'; '7c87'; '4ce4'; '5cc5'; '2c22'; '3c03'; '0c60'; '1c41';
	'edae'; 'fd8f'; 'cdec'; 'ddcd'; 'ad2a'; 'bd0b'; '8d68'; '9d49';
	'7e97'; '6eb6'; '5ed5'; '4ef4'; '3e13'; '2e32'; '1e51'; '0e70';
	'ff9f'; 'efbe'; 'dfdd'; 'cffc'; 'bf1b'; 'af3a'; '9f59'; '8f78';
	'9188'; '81a9'; 'b1ca'; 'a1eb'; 'd10c'; 'c12d'; 'f14e'; 'e16f';
	'1080'; '00a1'; '30c2'; '20e3'; '5004'; '4025'; '7046'; '6067';
	'83b9'; '9398'; 'a3fb'; 'b3da'; 'c33d'; 'd31c'; 'e37f'; 'f35e';
	'02b1'; '1290'; '22f3'; '32d2'; '4235'; '5214'; '6277'; '7256';
	'b5ea'; 'a5cb'; '95a8'; '8589'; 'f56e'; 'e54f'; 'd52c'; 'c50d';
	'34e2'; '24c3'; '14a0'; '0481'; '7466'; '6447'; '5424'; '4405';
	'a7db'; 'b7fa'; '8799'; '97b8'; 'e75f'; 'f77e'; 'c71d'; 'd73c';
	'26d3'; '36f2'; '0691'; '16b0'; '6657'; '7676'; '4615'; '5634';
	'd94c'; 'c96d'; 'f90e'; 'e92f'; '99c8'; '89e9'; 'b98a'; 'a9ab';
	'5844'; '4865'; '7806'; '6827'; '18c0'; '08e1'; '3882'; '28a3';
	'cb7d'; 'db5c'; 'eb3f'; 'fb1e'; '8bf9'; '9bd8'; 'abbb'; 'bb9a';
	'4a75'; '5a54'; '6a37'; '7a16'; '0af1'; '1ad0'; '2ab3'; '3a92';
	'fd2e'; 'ed0f'; 'dd6c'; 'cd4d'; 'bdaa'; 'ad8b'; '9de8'; '8dc9';
	'7c26'; '6c07'; '5c64'; '4c45'; '3ca2'; '2c83'; '1ce0'; '0cc1';
	'ef1f'; 'ff3e'; 'cf5d'; 'df7c'; 'af9b'; 'bfba'; '8fd9'; '9ff8';
	'6e17'; '7e36'; '4e55'; '5e74'; '2e93'; '3eb2'; '0ed1'; '1ef0';
]));

% Message size
crc_Hils = uint16(0);
data = zeros(10,1);

% Check if the packet has correct header
if ((packet(1) == 126) && (packet(2) == 129))
    % Confirmed the header is correct, proceed to check CRC
    for i=3:22
        datain = bitand(uint16(packet(i)), hex2dec('00FF'));
        crcidx = bitxor(bitshift(crc_Hils, -8, 'uint16'), datain, 'uint16');
        crcidx_temp = bitand(crcidx, hex2dec('00FF'), 'uint16');
        crc_Hils = bitxor(bitshift(crc_Hils, 8, 'uint16'), crc_table(crcidx_temp+1), 'uint16');        
    end
    if (crc_Hils == 0)
        % Packet decode
        data(1,1) = packet(3);  % Length 
        data(2,1) = RxFloat32(packet(4), packet(5), packet(6), packet(7));  % Time
        data(3,1) = RxUint16(packet(8) , packet(9));     % mag_moment X
        data(4,1) = RxUint16(packet(10), packet(11));    % mag_moment Y
        data(5,1) = RxUint16(packet(12), packet(13));    % mag_moment Z
        data(6,1) = RxUint16(packet(14), packet(15));    % TRIAD angle X
        data(7,1) = RxUint16(packet(16), packet(17));    % TRIAD angle Y
        data(8,1) = RxUint16(packet(18), packet(19));    % TRIAD angle Z
        data(9,1) = 1; % Dummy
        data(10,1) = 1; % Dummy
    else
        data(1,1) = 1;
        data(2,1) = 2;
        data(3,1) = 3;
        data(4,1) = 4;
        data(5,1) = 5;
        data(6,1) = 6;
        data(7,1) = 6;
        data(8,1) = 8;
        data(9,1) = 9;
        data(10,1) = 10;
    end
end
end

function Out = RxFloat32(byte1, byte2, byte3, byte4)
dummy1 = bitor(bitshift(cast(byte4, 'uint32'), 24, 'uint32'), ...
               bitshift(cast(byte3, 'uint32'), 16, 'uint32'));
dummy2 = bitor(bitshift(cast(byte2, 'uint32'), 8, 'uint32'), ...
               cast(byte1, 'uint32'));
dummy3 = bitor(dummy1, dummy2, 'uint32');
dummy4 = typecast(dummy3, 'single');
Out = double(dummy4);
end

function Out = RxUint16(MSB, LSB)
Out = bitor(bitshift(cast(MSB,'uint16'), 8, 'uint16'), cast(LSB, 'uint16'), 'uint16');
end
